simulink model "test_flowsensing_inout"  (R2022b)
settings: Solver=VariableStepAuto  StartTime=0.0  StopTime=10.0  RelTol=1e-3
undefined symbols (not defined in the file): CustomValue, FaultMode, MinVcc, Vcc
libraries: simulink x1, hil_flowsensing_lib x1
settings Model: Creator=CentoPas  LastModifiedBy=Km
settings SolverCC: AlgebraicLoopSolver=TrustRegion
settings OptimizationCC: DefaultParameterBehavior=Inlined  EnhancedBackFolding=on  PassReuseOutputArgsAs=Individual arguments  ZeroExternalMemoryAtStartup=off  ZeroInternalMemoryAtStartup=off  OptimizeBlockOrder=speed  DifferentSizesBufferReuse=on  OptimizationCustomize=off  EfficientTunableParamExpr=on
settings DebuggingCC: ParameterTunabilityLossMsg=error  UnconnectedInputMsg=warning  UnconnectedOutputMsg=warning  UnconnectedLineMsg=warning  SFMachineParentedDataDiag=warning
settings ModelReferenceCC: EnableRefExpFcnMdlSchedulingChecks=on
settings SFSimCC: SimGenImportedTypeDefs=on  MATLABDynamicMemAlloc=off
settings RTWCC: Description=Embedded Coder  SystemTargetFile=ert.tlc  TemplateMakefile=ert_default_tmf
settings CodeAppCC: ForceParamTrailComments=on  IgnoreCustomStorageClasses=off  OperatorAnnotations=on  SimulinkDataObjDesc=on  SFDataObjDesc=on  InsertBlockDesc=on
settings ERTTargetCC: TargetLangStandard=C99 (ISO)  GenerateSampleERTMain=on  InlinedParameterPlacement=NonHierarchical  ERTCustomFileTemplate=example_file_process.tlc

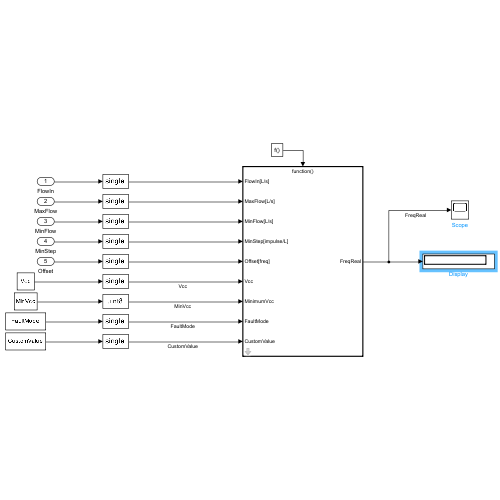
[thumbnail: Simulink's stored preview of the top-level diagram]
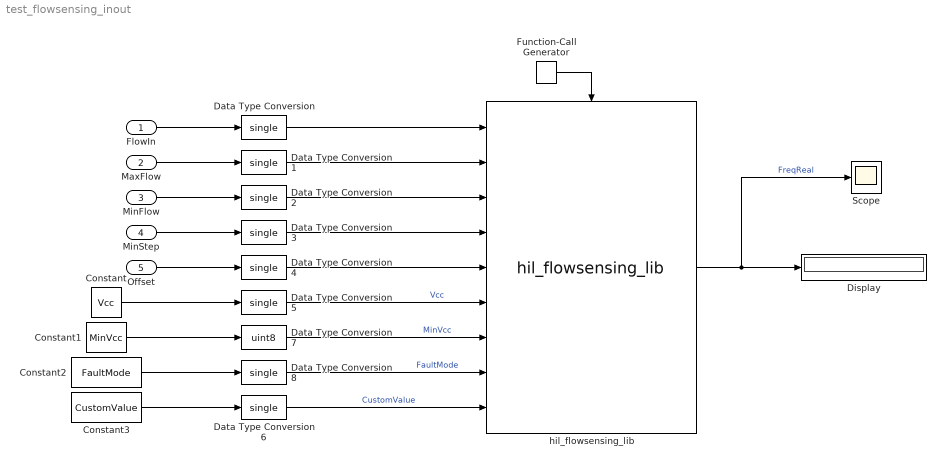
== system test_flowsensing_inout ==
  FlowIn : Inport
  MaxFlow : Inport  Port=2
  MinFlow : Inport  Port=3
  MinStep : Inport  Port=4
  Offset : Inport  Port=5
  Constant : Constant  Value=Vcc
  Constant1 : Constant  Value=MinVcc
  Constant2 : Constant  Value=FaultMode
  Constant3 : Constant  Value=CustomValue
  Data Type Conversion{,1..6,8} (8 alike) : DataTypeConversion  OutDataTypeStr=single  SaturateOnIntegerOverflow=off  RndMeth=Floor
  Data Type Conversion7 : DataTypeConversion  OutDataTypeStr=uint8  SaturateOnIntegerOverflow=off  RndMeth=Floor
  Display : Display
  Function-Call Generator : simulink/Ports & Subsystems/Function-Call Generator  sample_time=0.001  numberOfIterations=1  DisallowWideOutput=off
  Scope : Scope
  hil_flowsensing_lib : hil_flowsensing_lib/hil_flowsensing_lib
  wires:
  Data Type Conversion/1 -> hil_flowsensing_lib/1
  MaxFlow/1 -> Data Type Conversion1/1
  MinFlow/1 -> Data Type Conversion2/1
  Data Type Conversion2/1 -> hil_flowsensing_lib/3
  MinStep/1 -> Data Type Conversion3/1
  Data Type Conversion3/1 -> hil_flowsensing_lib/4
  Offset/1 -> Data Type Conversion4/1
  Constant/1 -> Data Type Conversion5/1
  Constant3/1 -> Data Type Conversion6/1
  Constant1/1 -> Data Type Conversion7/1
  Data Type Conversion7/1 -> hil_flowsensing_lib/7  "MinVcc"
  hil_flowsensing_lib/1 -> Display/1, Scope/1  "FreqReal"
  Function-Call Generator/1 -> hil_flowsensing_lib/Trigger
  Data Type Conversion1/1 -> hil_flowsensing_lib/2
  Data Type Conversion4/1 -> hil_flowsensing_lib/5
  Constant2/1 -> Data Type Conversion8/1
  Data Type Conversion5/1 -> hil_flowsensing_lib/6  "Vcc"
  Data Type Conversion8/1 -> hil_flowsensing_lib/8  "FaultMode"
  Data Type Conversion6/1 -> hil_flowsensing_lib/9  "CustomValue"
  FlowIn/1 -> Data Type Conversion/1
